simulink subsystem "Thrust_to_RPM_MDL"  (R2024b)
settings: Solver=VariableStepAuto  StartTime=0.0  StopTime=10.0  RelTol=1e-3
undefined symbols (not defined in the file): SimIn
libraries: simulink x1
settings Model: Creator=bmsimmon  LastModifiedBy=macheson
settings RTWCC: GPUComputeCapability=3.5

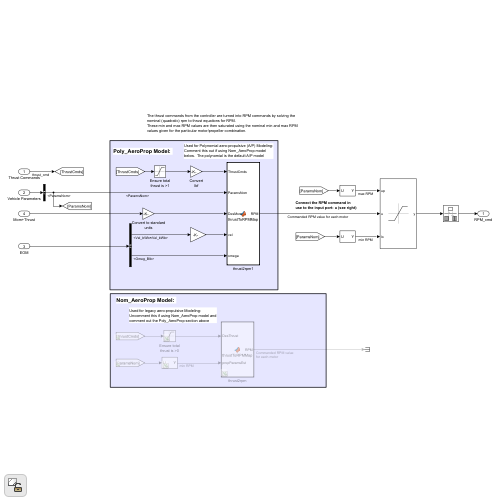
[thumbnail: Simulink's stored preview of the top-level diagram]
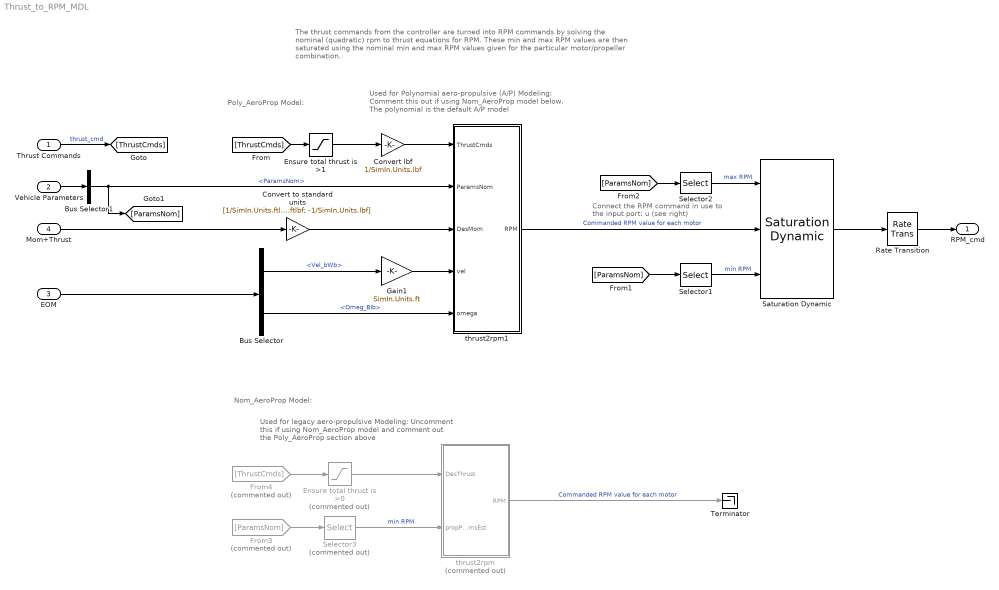
== system Thrust_to_RPM_MDL ==
  note: Connect the RPM command in
      | use to the input port: u (see right)
  note: Nom_AeroProp Model:
  note: Used for legacy aero-propulsive Modeling:
      | Uncomment this if using Nom_AeroProp model and
      | comment out the Poly_AeroProp section above
  note: The thrust commands from the controller are turned into RPM commands by solving the
      | nominal (quadratic) rpm to thrust equations for RPM.
      | These min and max RPM values are then saturated using the nominal min and max RPM
      | values given for the particular motor/propeller combination.
  note: Used for Polynomial aero-propulsive (A/P) Modeling:
      | Comment this out if using Nom_AeroProp model
      | below.  The polynomial is the default A/P model
  note: Poly_AeroProp Model:
  Thrust Commands : Inport
  Vehicle Parameters : Inport  Port=2
  EOM : Inport  Port=3
  Mom+Thrust : Inport  Port=4
  Bus Selector : BusSelector  OutputSignals=AirRelativeData.Vel_bWb,InertialData.Omeg_BIb
  Bus Selector1 : BusSelector  OutputSignals=ParamsNom
  Convert lbf : Gain  Gain=1/SimIn.Units.lbf
  Convert to standard units : Gain  Gain=[1/SimIn.Units.ftlbf; 1/SimIn.Units.ftlbf; 1/SimIn.Units.ftlbf; -1/SimIn.Units.lbf]
  Ensure total thrust is >0 : Saturate  Commented=on  UpperLimit=inf  LowerLimit=0
  Ensure total thrust is >1 : Saturate  UpperLimit=inf  LowerLimit=0
  From3 : From  Commented=on  GotoTag=ParamsNom
  From4 : From  Commented=on  GotoTag=ThrustCmds
  Gain1 : Gain  Gain=SimIn.Units.ft
  Rate Transition : RateTransition  OutPortSampleTime=SimIn.FCS.t_control
  Saturation Dynamic : simulink/Discontinuities/Saturation Dynamic  OutMin=[]  OutMax=[]  OutDataTypeStr=Inherit: Same as second input  OutDataType=fixdt(1, 16)  OutScaling=2^-10  DoSatur=off
  Selector1 : Selector  NumberOfDimensions=2  InputPortWidth=17  IndexOptions=Select all,Index vector (dialog)  Indices=11,11  OutputSizes=1,1
  Selector2 : Selector  NumberOfDimensions=2  InputPortWidth=17  IndexOptions=Select all,Index vector (dialog)  Indices=[12],12  OutputSizes=1,1
  Selector3 : Selector  Commented=on  NumberOfDimensions=2  InputPortWidth=17  IndexOptions=Select all,Index vector (dialog)  Indices=11,[7 8]  OutputSizes=1,1
  Terminator : Terminator
  thrust2rpm : MATLAB Function  Commented=on  TreatAsAtomicUnit=on
  thrust2rpm1 : MATLAB Function  TreatAsAtomicUnit=on
  RPM_cmd : Outport  VectorParamsAs1DForOutWhenUnconnected=off
  wires:
  Vehicle Parameters/1 -> Bus Selector1/1
  Ensure total thrust is >0/1 -> thrust2rpm/1(DesThrust)
  Selector2/1 -> Saturation Dynamic/1  "max RPM"
  Saturation Dynamic/1 -> Rate Transition/1
  Selector1/1 -> Saturation Dynamic/3  "min RPM"
  Rate Transition/1 -> RPM_cmd/1
  EOM/1 -> Bus Selector/1
  Bus Selector/1 -> Gain1/1  "<Vel_bWb>"
  thrust2rpm1/1(RPM) -> Saturation Dynamic/2  "Commanded RPM value for each motor"
  Selector3/1 -> thrust2rpm/2(propParamsEst)  "min RPM"
  Bus Selector/2 -> thrust2rpm1/5(omega)  "<Omeg_BIb>"
  Mom+Thrust/1 -> Convert to standard units/1
  Convert to standard units/1 -> thrust2rpm1/3(DesMom)
  Gain1/1 -> thrust2rpm1/4(vel)
  [ThrustCmds] -> Ensure total thrust is >1/1
  Convert lbf/1 -> thrust2rpm1/1(ThrustCmds)
  Ensure total thrust is >1/1 -> Convert lbf/1
  Bus Selector1/1 -> [ParamsNom], thrust2rpm1/2(ParamsNom)  "<ParamsNom>"
  [ParamsNom] -> Selector1/1
  [ParamsNom] -> Selector2/1
  From3/1 -> Selector3/1
  Thrust Commands/1 -> [ThrustCmds]  "thrust_cmd"
  From4/1 -> Ensure total thrust is >0/1
  thrust2rpm/1(RPM) -> Terminator/1  "Commanded RPM value for each motor"

== matlab function Thrust_to_RPM_MDL/thrust2rpm ==
  data: DesThrust input; RPM output; propParamsEst input
function RPM = thrustToRPMMap(DesThrust, propParamsEst)

RPM = Thrust2RpmPolyMdl(DesThrust, propParamsEst);

== matlab function Thrust_to_RPM_MDL/thrust2rpm1 ==
  data: ThrustCmds input; ParamsNom input; DesMom input; RPM output; vel input; omega input
function RPM = thrustToRPMMap(ThrustCmds, ParamsNom, DesMom, vel, omega)

RPM = Thrust2RpmPolyMdl_Impact(ThrustCmds, ParamsNom, DesMom, vel, omega);
